simulink model "Target_Control_System"  (R2021b)
settings: Solver=FixedStepDiscrete  StartTime=0.0  StopTime=5  RelTol=1e-3
PreLoadFcn:
  | RTWConfigurationCB('preloadfcn', bdroot);
PostLoadFcn:
  | load('configuration/data_struct.mat');
  | load('configuration/fluxMaps_propMotor.mat');
  | load('configuration/parameterInit_PROP.mat');
  | load('configuration/parameterInit_PUMP.mat');
  | load('configuration/parameterInit_PITCH.mat');
  | load('configuration/parameterInit_TILT.mat');
  | %load('configuration/base_workspace_signal_definition.mat');
  | %load('resolvedatastores_to_baseworkspace_for_faster_simulation.mat');
model workspace (MAT data in the model file):
  SIMULATION_OPTIONS : Simulink.Parameter (value not decoded)
  TARGET_CODE_GEN : Simulink.Parameter (value not decoded)
  TCS_SAMPLE_FREQ_HZ : Simulink.Parameter (value not decoded)
symbols that are objects in the model workspace (value not decoded): TARGET_CODE_GEN, TCS_SAMPLE_FREQ_HZ
undefined symbols (not defined in the file): A_DQ_REF_LPF_INIT__PITCH, A_DQ_REF_LPF_INIT__PROP, A_DQ_REF_LPF_INIT__PUMP, A_DQ_REF_LPF_INIT__TILT, A_OBSERVER_CONFIDENCE_INIT__PITCH, A_OBSERVER_CONFIDENCE_INIT__PROP, A_OBSERVER_CONFIDENCE_INIT__PUMP, A_OBSERVER_CONFIDENCE_INIT__TILT, ACTUATOR_MAX_ANGLE_TRIP__PITCH, ACTUATOR_MIN_ANGLE_TRIP__PITCH, ACTUATOR_POS_SENSOR_INV_DIRECTION__PITCH, ACTUATOR_POS_SENSOR_INV_DIRECTION__TILT, ACTUATOR_POS_SENSOR_OFFSET__PITCH, ACTUATOR_POS_SENSOR_OFFSET__TILT, ADC_scaler1_baseaddr_TILT, ADC_SCALER_FLOAT_TO_FIXPOINT_EXPANSION, ANGLE_ELEC_FROM_SENSOR_OFFSET_INIT__PITCH, ANGLE_ELEC_FROM_SENSOR_OFFSET_INIT__PROP, ANGLE_ELEC_FROM_SENSOR_OFFSET_INIT__PUMP, ANGLE_ELEC_FROM_SENSOR_OFFSET_INIT__TILT, AUTO_CLEAR_FAULTS_ENABLED__PITCH, AUTO_CLEAR_FAULTS_ENABLED__PROP, AUTO_CLEAR_FAULTS_ENABLED__PUMP, AUTO_CLEAR_FAULTS_ENABLED__TILT, AUTO_CLEAR_FAULTS_WAIT_TICKS__PITCH, AUTO_CLEAR_FAULTS_WAIT_TICKS__PROP, AUTO_CLEAR_FAULTS_WAIT_TICKS__PUMP, AUTO_CLEAR_FAULTS_WAIT_TICKS__TILT, AUTO_I_ZERO_IDLE_TICKS__PITCH, AUTO_I_ZERO_IDLE_TICKS__PROP, AUTO_I_ZERO_IDLE_TICKS__PUMP, AUTO_I_ZERO_IDLE_TICKS__TILT, AUTO_I_ZERO_OFFSET_IDC_THRESHOLD__PITCH, AUTO_I_ZERO_OFFSET_IDC_THRESHOLD__PROP, AUTO_I_ZERO_OFFSET_IDC_THRESHOLD__PUMP, AUTO_I_ZERO_OFFSET_IDC_THRESHOLD__TILT, AUTO_I_ZERO_OFFSET_IPH_THRESHOLD__PITCH, AUTO_I_ZERO_OFFSET_IPH_THRESHOLD__PROP, AUTO_I_ZERO_OFFSET_IPH_THRESHOLD__PUMP, AUTO_I_ZERO_OFFSET_IPH_THRESHOLD__TILT, AUTO_SENSORLESS_SWITCHOVER_DISABLE_OMEGA, AUTO_SENSORLESS_SWITCHOVER_ENABLE_OMEGA, AUTO_SENSORLESS_SWITCHOVER_MIN_CONFIDENCE, AUXILIARY_PROTECTION_UNIT_BASEADDR__TILT, blanking_max_error_omega_INIT_PITCH, blanking_max_error_omega_INIT_TILT, blanking_max_error_position_INIT_PITCH, blanking_max_error_position_INIT_TILT, BRUTE_START_I_Q_REF_RAMP_SPEED__PITCH, BRUTE_START_I_Q_REF_RAMP_SPEED__PROP, BRUTE_START_I_Q_REF_RAMP_SPEED__PUMP, BRUTE_START_I_Q_REF_RAMP_SPEED__TILT, CONTROL_LOOP_DT_INIT__PITCH, CONTROL_LOOP_DT_INIT__PROP, CONTROL_LOOP_DT_INIT__PUMP, CONTROL_LOOP_DT_INIT__TILT, CORRECTION_FILTER_SCALE__PITCH, CORRECTION_FILTER_SCALE__PROP, CORRECTION_FILTER_SCALE__PUMP, CORRECTION_FILTER_SCALE__TILT ... (+458)
libraries: simulink x178, Reusables_Lib x24
(part 4 of 47)

== system Target_Control_System/Target_Control_System/InterruptFunction/pumpMotor_dataToIsr ==
  motorDataFromMainToIsr : TriggerPort  TriggerType=function-call  VariantControl=Variant
  Data Store Read : DataStoreRead  DataStoreName=oPump  DataStoreElements=oPump.oMot_.oOut_.fOneOverUdc_  IndexOptions=Index vector (dialog)  Indices=1  OutputSizes=1
  Data Store Read1 : DataStoreRead  DataStoreName=oPump  DataStoreElements=oPump.oMot_.oState_.oRampDataOmegaERef_.fRampOut_  IndexOptions=Index vector (dialog)  Indices=1  OutputSizes=1
  Data Store Read10 : DataStoreRead  DataStoreName=oPump  DataStoreElements=oPump.oMot_.oOut_.uiCurrentControllerActive_  IndexOptions=Index vector (dialog)  Indices=1  OutputSizes=1
  Data Store Read11 : DataStoreRead  DataStoreName=oPump  DataStoreElements=oPump.oMot_.oState_.oRampDataFluxFeedforwardGain_.fRampOut_  IndexOptions=Index vector (dialog)  Indices=1  OutputSizes=1
  Data Store Read12 : DataStoreRead  DataStoreName=oPump  DataStoreElements=oPump.oMot_.oState_.uiDriveState_  IndexOptions=Index vector (dialog)  Indices=1  OutputSizes=1
  Data Store Read13 : DataStoreRead  DataStoreName=oPump  DataStoreElements=oPump.oMot_.oOut_.uiPwmRequestFromMain_  IndexOptions=Index vector (dialog)  Indices=1  OutputSizes=1
  Data Store Read14 : DataStoreRead  DataStoreName=oPump  DataStoreElements=oPump.oMot_.oOut_.uiPwmDutyTicksFromMainA_  IndexOptions=Index vector (dialog)  Indices=1  OutputSizes=1
  Data Store Read15 : DataStoreRead  DataStoreName=oPump  DataStoreElements=oPump.oMot_.oOut_.uiPwmDutyTicksFromMainB_  IndexOptions=Index vector (dialog)  Indices=1  OutputSizes=1
  Data Store Read16 : DataStoreRead  DataStoreName=oPump  DataStoreElements=oPump.oMot_.oOut_.uiPwmDutyTicksFromMainC_  IndexOptions=Index vector (dialog)  Indices=1  OutputSizes=1
  Data Store Read17 : DataStoreRead  DataStoreName=oPump  DataStoreElements=oPump.oMot_.oState_.oPosSensor_.fAngleElecFromSensor_  IndexOptions=Index vector (dialog)  Indices=1  OutputSizes=1
  Data Store Read18 : DataStoreRead  DataStoreName=oPump  DataStoreElements=oPump.oMot_.oState_.oPosSensor_.fOmegaEFromSensor_  IndexOptions=Index vector (dialog)  Indices=1  OutputSizes=1
  Data Store Read2 : DataStoreRead  DataStoreName=oPump  DataStoreElements=oPump.oMot_.oState_.oRampDataFluxMasterAngleOffset_.fRampOut_  IndexOptions=Index vector (dialog)  Indices=1  OutputSizes=1
  Data Store Read3 : DataStoreRead  DataStoreName=oPump  DataStoreElements=oPump.oMot_.oState_.oRampDataIqRef_.fRampOut_  IndexOptions=Index vector (dialog)  Indices=1  OutputSizes=1
  Data Store Read4 : DataStoreRead  DataStoreName=oPump  DataStoreElements=oPump.oMot_.oState_.oRampDataIdRef_.fRampOut_  IndexOptions=Index vector (dialog)  Indices=1  OutputSizes=1
  Data Store Read5 : DataStoreRead  DataStoreName=oPump  DataStoreElements=oPump.oMot_.oParam_.fIdRefFractionOfIq_  IndexOptions=Index vector (dialog)  Indices=1  OutputSizes=1
  Data Store Read6 : DataStoreRead  DataStoreName=oPump  DataStoreElements=oPump.oMot_.oOut_.fUphFilterAmplitudeRatio_  IndexOptions=Index vector (dialog)  Indices=1  OutputSizes=1
  Data Store Read7 : DataStoreRead  DataStoreName=oPump  DataStoreElements=oPump.oMot_.oOut_.fUphFilterDelayAngleRad_  IndexOptions=Index vector (dialog)  Indices=1  OutputSizes=1
  Data Store Read8 : DataStoreRead  DataStoreName=oPump  DataStoreElements=oPump.oMot_.oState_.oRampDataFluxMstrAngFrcd2clsdSmoothn_.fRampOut_  IndexOptions=Index vector (dialog)  Indices=1  OutputSizes=1
  Data Store Read9 : DataStoreRead  DataStoreName=oPump  DataStoreElements=oPump.oMot_.oOut_.uiForcedAngle_  IndexOptions=Index vector (dialog)  Indices=1  OutputSizes=1
  Data Store Write1 : DataStoreWrite  DataStoreName=oPump  DataStoreElements=oPump.oIsr_.oIn_.fOneOverUdc_  IndexOptions=Index vector (dialog)  Indices=1  OutputSizes=1
  Data Store Write10 : DataStoreWrite  DataStoreName=oPump  DataStoreElements=oPump.oIsr_.oIn_.uiForcedAngle_  IndexOptions=Index vector (dialog)  Indices=1  OutputSizes=1
  Data Store Write11 : DataStoreWrite  DataStoreName=oPump  DataStoreElements=oPump.oIsr_.oIn_.uiCurrentControllerActive_  IndexOptions=Index vector (dialog)  Indices=1  OutputSizes=1
  Data Store Write12 : DataStoreWrite  DataStoreName=oPump  DataStoreElements=oPump.oIsr_.oIn_.fFluxFeedforwardGainRampOut_  IndexOptions=Index vector (dialog)  Indices=1  OutputSizes=1
  Data Store Write13 : DataStoreWrite  DataStoreName=oPump  DataStoreElements=oPump.oIsr_.oIn_.uiDriveState_  IndexOptions=Index vector (dialog)  Indices=1  OutputSizes=1
  Data Store Write14 : DataStoreWrite  DataStoreName=oPump  DataStoreElements=oPump.oIsr_.oIn_.uiPwmRequestFromMain_  IndexOptions=Index vector (dialog)  Indices=1  OutputSizes=1
  Data Store Write15 : DataStoreWrite  DataStoreName=oPump  DataStoreElements=oPump.oIsr_.oIn_.uiPwmDutyTicksFromMainA_  IndexOptions=Index vector (dialog)  Indices=1  OutputSizes=1
  Data Store Write16 : DataStoreWrite  DataStoreName=oPump  DataStoreElements=oPump.oIsr_.oIn_.uiPwmDutyTicksFromMainB_  IndexOptions=Index vector (dialog)  Indices=1  OutputSizes=1
  Data Store Write17 : DataStoreWrite  DataStoreName=oPump  DataStoreElements=oPump.oIsr_.oIn_.uiPwmDutyTicksFromMainC_  IndexOptions=Index vector (dialog)  Indices=1  OutputSizes=1
  Data Store Write18 : DataStoreWrite  DataStoreName=oPump  DataStoreElements=oPump.oIsr_.oIn_.fAngleElecFromPosSensor_  IndexOptions=Index vector (dialog)  Indices=1  OutputSizes=1
  Data Store Write19 : DataStoreWrite  DataStoreName=oPump  DataStoreElements=oPump.oIsr_.oIn_.fOmegaElecFromPosSensor_  IndexOptions=Index vector (dialog)  Indices=1  OutputSizes=1
  Data Store Write2 : DataStoreWrite  DataStoreName=oPump  DataStoreElements=oPump.oIsr_.oIn_.fOmegaERefRampOut_  IndexOptions=Index vector (dialog)  Indices=1  OutputSizes=1
  Data Store Write3 : DataStoreWrite  DataStoreName=oPump  DataStoreElements=oPump.oIsr_.oIn_.fFluxMasterAngleOffsetRampOut_  IndexOptions=Index vector (dialog)  Indices=1  OutputSizes=1
  Data Store Write4 : DataStoreWrite  DataStoreName=oPump  DataStoreElements=oPump.oIsr_.oIn_.fIqRefRampOut_  IndexOptions=Index vector (dialog)  Indices=1  OutputSizes=1
  Data Store Write5 : DataStoreWrite  DataStoreName=oPump  DataStoreElements=oPump.oIsr_.oIn_.fIdRefRampOut_  IndexOptions=Index vector (dialog)  Indices=1  OutputSizes=1
  Data Store Write6 : DataStoreWrite  DataStoreName=oPump  DataStoreElements=oPump.oIsr_.oIn_.fIdRefFractionOfIq_  IndexOptions=Index vector (dialog)  Indices=1  OutputSizes=1
  Data Store Write7 : DataStoreWrite  DataStoreName=oPump  DataStoreElements=oPump.oIsr_.oIn_.fUphFilterAmplitudeRatio_  IndexOptions=Index vector (dialog)  Indices=1  OutputSizes=1
  Data Store Write8 : DataStoreWrite  DataStoreName=oPump  DataStoreElements=oPump.oIsr_.oIn_.fUphFilterDelayAngleRad_  IndexOptions=Index vector (dialog)  Indices=1  OutputSizes=1
  Data Store Write9 : DataStoreWrite  DataStoreName=oPump  DataStoreElements=oPump.oIsr_.oIn_.fFluxMasterAngleForced2closedSmoothingRampOut_  IndexOptions=Index vector (dialog)  Indices=1  OutputSizes=1
  wires:
  Data Store Read2/1 -> Data Store Write3/1
  Data Store Read12/1 -> Data Store Write13/1
  Data Store Read13/1 -> Data Store Write14/1
  Data Store Read16/1 -> Data Store Write17/1
  Data Store Read5/1 -> Data Store Write6/1
  Data Store Read10/1 -> Data Store Write11/1
  Data Store Read/1 -> Data Store Write1/1
  Data Store Read14/1 -> Data Store Write15/1
  Data Store Read8/1 -> Data Store Write9/1
  Data Store Read9/1 -> Data Store Write10/1
  Data Store Read3/1 -> Data Store Write4/1
  Data Store Read7/1 -> Data Store Write8/1
  Data Store Read11/1 -> Data Store Write12/1
  Data Store Read15/1 -> Data Store Write16/1
  Data Store Read17/1 -> Data Store Write18/1
  Data Store Read1/1 -> Data Store Write2/1
  Data Store Read18/1 -> Data Store Write19/1
  Data Store Read4/1 -> Data Store Write5/1
  Data Store Read6/1 -> Data Store Write7/1

== system Target_Control_System/Target_Control_System/InterruptFunction/pumpMotor_dataToMain ==
  motorDataFromIsrToMain : TriggerPort  TriggerType=function-call  VariantControl=Variant
  Constant : Constant  OutDataTypeStr=uint32  SampleTime=-1
  Data Store Read : DataStoreRead  DataStoreName=oPump  DataStoreElements=oPump.oIsr_.oOut_.fPowerDc_  IndexOptions=Index vector (dialog)  Indices=1  OutputSizes=1
  Data Store Read1 : DataStoreRead  DataStoreName=oPump  DataStoreElements=oPump.oIsr_.oOut_.fTEstimate_  IndexOptions=Index vector (dialog)  Indices=1  OutputSizes=1
  Data Store Read10 : DataStoreRead  DataStoreName=oPump  DataStoreElements=oPump.oIsr_.oState_.fUdRef_  IndexOptions=Index vector (dialog)  Indices=1  OutputSizes=1
  Data Store Read11 : DataStoreRead  DataStoreName=oPump  DataStoreElements=oPump.oIsr_.oState_.fFluxMasterAngle_  IndexOptions=Index vector (dialog)  Indices=1  OutputSizes=1
  Data Store Read12 : DataStoreRead  DataStoreName=oPump  DataStoreElements=oPump.oIsr_.oState_.fSoftILimitActual_  IndexOptions=Index vector (dialog)  Indices=1  OutputSizes=1
  Data Store Read13 : DataStoreRead  DataStoreName=oPump  DataStoreElements=oPump.oIsr_.oState_.fFluxMainAngleRaw2_  IndexOptions=Index vector (dialog)  Indices=1  OutputSizes=1
  Data Store Read14 : DataStoreRead  DataStoreName=oPump  DataStoreElements=oPump.oIsr_.oState_.fRMeasured_  IndexOptions=Index vector (dialog)  Indices=1  OutputSizes=1
  Data Store Read15 : DataStoreRead  DataStoreName=oPump  DataStoreElements=oPump.oIsr_.oOut_.uiPwmSetByIsr_  IndexOptions=Index vector (dialog)  Indices=1  OutputSizes=1
  Data Store Read16 : DataStoreRead  DataStoreName=oPump  DataStoreElements=oPump.oIsr_.oIn_.oAdcData_.fIa_  IndexOptions=Index vector (dialog)  Indices=1  OutputSizes=1
  Data Store Read17 : DataStoreRead  DataStoreName=oPump  DataStoreElements=oPump.oIsr_.oIn_.oAdcData_.fIb_  IndexOptions=Index vector (dialog)  Indices=1  OutputSizes=1
  Data Store Read18 : DataStoreRead  DataStoreName=oPump  DataStoreElements=oPump.oIsr_.oIn_.oAdcData_.fIc_  IndexOptions=Index vector (dialog)  Indices=1  OutputSizes=1
  Data Store Read19 : DataStoreRead  DataStoreName=oPump  DataStoreElements=oPump.oIsr_.oIn_.oAdcData_.fIdc_  IndexOptions=Index vector (dialog)  Indices=1  OutputSizes=1
  Data Store Read2 : DataStoreRead  DataStoreName=oPump  DataStoreElements=oPump.oIsr_.oOut_.fIPhaseMagnitude_  IndexOptions=Index vector (dialog)  Indices=1  OutputSizes=1
  Data Store Read20 : DataStoreRead  DataStoreName=oPump  DataStoreElements=oPump.oIsr_.oOut_.fUdc_  IndexOptions=Index vector (dialog)  Indices=1  OutputSizes=1
  Data Store Read21 : DataStoreRead  DataStoreName=oPump  DataStoreElements=oPump.oIsr_.oIn_.oAdcData_.fMotorEncoderFloat_  IndexOptions=Index vector (dialog)  Indices=1  OutputSizes=1
  Data Store Read22 : DataStoreRead  DataStoreName=oPump  DataStoreElements=oPump.oIsr_.oIn_.oAdcData_.fOutputEncoderFloat_  IndexOptions=Index vector (dialog)  Indices=1  OutputSizes=1
  Data Store Read23 : DataStoreRead  DataStoreName=oPump  DataStoreElements=oPump.oIsr_.oIn_.oAdcData_.fMotorSensorSpeed_  IndexOptions=Index vector (dialog)  Indices=1  OutputSizes=1
  Data Store Read3 : DataStoreRead  DataStoreName=oPump  DataStoreElements=oPump.oIsr_.oState_.fFluxMainMagnitudeLpf_  IndexOptions=Index vector (dialog)  Indices=1  OutputSizes=1
  Data Store Read4 : DataStoreRead  DataStoreName=oPump  DataStoreElements=oPump.oIsr_.oState_.fOmegaEObserverLpf2_  IndexOptions=Index vector (dialog)  Indices=1  OutputSizes=1
  Data Store Read5 : DataStoreRead  DataStoreName=oPump  DataStoreElements=oPump.oIsr_.oState_.fOmegaEObserverRaw2_  IndexOptions=Index vector (dialog)  Indices=1  OutputSizes=1
  Data Store Read6 : DataStoreRead  DataStoreName=oPump  DataStoreElements=oPump.oIsr_.oState_.fId_  IndexOptions=Index vector (dialog)  Indices=1  OutputSizes=1
  Data Store Read7 : DataStoreRead  DataStoreName=oPump  DataStoreElements=oPump.oIsr_.oState_.fIq_  IndexOptions=Index vector (dialog)  Indices=1  OutputSizes=1
  Data Store Read8 : DataStoreRead  DataStoreName=oPump  DataStoreElements=oPump.oIsr_.oState_.fIdRefTotal_  IndexOptions=Index vector (dialog)  Indices=1  OutputSizes=1
  Data Store Read9 : DataStoreRead  DataStoreName=oPump  DataStoreElements=oPump.oIsr_.oState_.fUqRef_  IndexOptions=Index vector (dialog)  Indices=1  OutputSizes=1
  Data Store Write1 : DataStoreWrite  DataStoreName=oPump  DataStoreElements=oPump.oMot_.oIn_.fPowerDc_  IndexOptions=Index vector (dialog)  Indices=1  OutputSizes=1
  Data Store Write10 : DataStoreWrite  DataStoreName=oPump  DataStoreElements=oPump.oMot_.oIn_.fUqRef_  IndexOptions=Index vector (dialog)  Indices=1  OutputSizes=1
  Data Store Write11 : DataStoreWrite  DataStoreName=oPump  DataStoreElements=oPump.oMot_.oIn_.fUdRef_  IndexOptions=Index vector (dialog)  Indices=1  OutputSizes=1
  Data Store Write12 : DataStoreWrite  DataStoreName=oPump  DataStoreElements=oPump.oMot_.oIn_.fFluxMasterAngle_  IndexOptions=Index vector (dialog)  Indices=1  OutputSizes=1
  Data Store Write13 : DataStoreWrite  DataStoreName=oPump  DataStoreElements=oPump.oMot_.oIn_.fSoftILimitActual_  IndexOptions=Index vector (dialog)  Indices=1  OutputSizes=1
  Data Store Write14 : DataStoreWrite  DataStoreName=oPump  DataStoreElements=oPump.oMot_.oIn_.fFluxMainAngleRaw2_  IndexOptions=Index vector (dialog)  Indices=1  OutputSizes=1
  Data Store Write15 : DataStoreWrite  DataStoreName=oPump  DataStoreElements=oPump.oMot_.oIn_.fRMeasured_  IndexOptions=Index vector (dialog)  Indices=1  OutputSizes=1
  Data Store Write16 : DataStoreWrite  DataStoreName=oPump  DataStoreElements=oPump.oMot_.oIn_.uiPwmSetByIsr_  IndexOptions=Index vector (dialog)  Indices=1  OutputSizes=1
  Data Store Write17 : DataStoreWrite  DataStoreName=oPump  DataStoreElements=oPump.oMot_.oIn_.oAdcData_.fIa_  IndexOptions=Index vector (dialog)  Indices=1  OutputSizes=1
  Data Store Write18 : DataStoreWrite  DataStoreName=oPump  DataStoreElements=oPump.oMot_.oIn_.oAdcData_.fIb_  IndexOptions=Index vector (dialog)  Indices=1  OutputSizes=1
  Data Store Write19 : DataStoreWrite  DataStoreName=oPump  DataStoreElements=oPump.oMot_.oIn_.oAdcData_.fIc_  IndexOptions=Index vector (dialog)  Indices=1  OutputSizes=1
  Data Store Write2 : DataStoreWrite  DataStoreName=oPump  DataStoreElements=oPump.oMot_.oIn_.fTEstimate_  IndexOptions=Index vector (dialog)  Indices=1  OutputSizes=1
  Data Store Write20 : DataStoreWrite  DataStoreName=oPump  DataStoreElements=oPump.oMot_.oIn_.oAdcData_.fIdc_  IndexOptions=Index vector (dialog)  Indices=1  OutputSizes=1
  Data Store Write21 : DataStoreWrite  DataStoreName=oPump  DataStoreElements=oPump.oMot_.oIn_.oAdcData_.fUdc_  IndexOptions=Index vector (dialog)  Indices=1  OutputSizes=1
  Data Store Write22 : DataStoreWrite  DataStoreName=oPump  DataStoreElements=oPump.oMot_.oIn_.oAdcData_.fMotorEncoderFloat_  IndexOptions=Index vector (dialog)  Indices=1  OutputSizes=1
  Data Store Write23 : DataStoreWrite  DataStoreName=oPump  DataStoreElements=oPump.oMot_.oIn_.oAdcData_.fOutputEncoderFloat_  IndexOptions=Index vector (dialog)  Indices=1  OutputSizes=1
  Data Store Write24 : DataStoreWrite  DataStoreName=oPump  DataStoreElements=oPump.oMot_.oIn_.oAdcData_.fMotorSensorSpeed_  IndexOptions=Index vector (dialog)  Indices=1  OutputSizes=1
  Data Store Write25 : DataStoreWrite  DataStoreName=oPump  DataStoreElements=oPump.oMot_.oIn_.uiDataFromIsrToMainUpdated_  IndexOptions=Index vector (dialog)  Indices=1  OutputSizes=1
  Data Store Write3 : DataStoreWrite  DataStoreName=oPump  DataStoreElements=oPump.oMot_.oIn_.fIPhaseMagnitude_  IndexOptions=Index vector (dialog)  Indices=1  OutputSizes=1
  Data Store Write4 : DataStoreWrite  DataStoreName=oPump  DataStoreElements=oPump.oMot_.oIn_.fFluxMainMagnitudeLpf_  IndexOptions=Index vector (dialog)  Indices=1  OutputSizes=1
  Data Store Write5 : DataStoreWrite  DataStoreName=oPump  DataStoreElements=oPump.oMot_.oIn_.fOmegaEObserverLpf2_  IndexOptions=Index vector (dialog)  Indices=1  OutputSizes=1
  Data Store Write6 : DataStoreWrite  DataStoreName=oPump  DataStoreElements=oPump.oMot_.oIn_.fOmegaEObserverRaw2_  IndexOptions=Index vector (dialog)  Indices=1  OutputSizes=1
  Data Store Write7 : DataStoreWrite  DataStoreName=oPump  DataStoreElements=oPump.oMot_.oIn_.fId_  IndexOptions=Index vector (dialog)  Indices=1  OutputSizes=1
  Data Store Write8 : DataStoreWrite  DataStoreName=oPump  DataStoreElements=oPump.oMot_.oIn_.fIq_  IndexOptions=Index vector (dialog)  Indices=1  OutputSizes=1
  Data Store Write9 : DataStoreWrite  DataStoreName=oPump  DataStoreElements=oPump.oMot_.oIn_.fIdRefTotal_  IndexOptions=Index vector (dialog)  Indices=1  OutputSizes=1
  wires:
  Data Store Read21/1 -> Data Store Write22/1
  Data Store Read19/1 -> Data Store Write20/1
  Data Store Read3/1 -> Data Store Write4/1
  Data Store Read20/1 -> Data Store Write21/1
  Data Store Read23/1 -> Data Store Write24/1
  Constant/1 -> Data Store Write25/1
  Data Store Read9/1 -> Data Store Write10/1
  Data Store Read22/1 -> Data Store Write23/1
  Data Store Read14/1 -> Data Store Write15/1
  Data Store Read7/1 -> Data Store Write8/1
  Data Store Read/1 -> Data Store Write1/1
  Data Store Read16/1 -> Data Store Write17/1
  Data Store Read10/1 -> Data Store Write11/1
  Data Store Read4/1 -> Data Store Write5/1
  Data Store Read12/1 -> Data Store Write13/1
  Data Store Read5/1 -> Data Store Write6/1
  Data Store Read8/1 -> Data Store Write9/1
  Data Store Read17/1 -> Data Store Write18/1
  Data Store Read2/1 -> Data Store Write3/1
  Data Store Read6/1 -> Data Store Write7/1
  Data Store Read13/1 -> Data Store Write14/1
  Data Store Read11/1 -> Data Store Write12/1
  Data Store Read1/1 -> Data Store Write2/1
  Data Store Read15/1 -> Data Store Write16/1
  Data Store Read18/1 -> Data Store Write19/1

== system Target_Control_System/Target_Control_System/InterruptFunction/pumpMotor_isrSchedule ==
  FunctionCallSchedulePump : TriggerPort  TriggerType=function-call  VariantControl=Variant
  Constant : Constant  OutDataTypeStr=uint32  SampleTime=-1
  Constant1 : Constant  Value=3  OutDataTypeStr=uint32  SampleTime=-1
  Data Store Read : DataStoreRead  DataStoreName=mdl_suiIsrSmallInvCounter_  IndexOptions=Index vector (dialog)  Indices=1  OutputSizes=1
  Equal : RelationalOperator  Operator===  OutDataTypeStr=boolean  RndMeth=Simplest
  Equal1 : RelationalOperator  Operator===  OutDataTypeStr=boolean  RndMeth=Simplest
  OR : Logic  Operator=OR  AllPortsSameDT=off  OutDataTypeStr=boolean
  Triggered Subsystem : Subsystem  TreatAsAtomicUnit=on
  Output : Outport
  wires:
  Constant1/1 -> Equal1/2
  Equal1/1 -> OR/2
  Constant/1 -> Equal/1
  Data Store Read/1 -> Equal1/1, Equal/2
  Equal/1 -> OR/1
  Triggered Subsystem/1(Output) -> Output/1
  OR/1 -> Triggered Subsystem/Trigger

== system Target_Control_System/Target_Control_System/InterruptFunction/pumpMotor_isrTask ==
  motorIntTaskStep : TriggerPort  TriggerType=function-call  VariantControl=Variant  PortDimensions=1
  Function-Call Generator : simulink/Ports & Subsystems/Function-Call Generator  sample_time=-1  numberOfIterations=1  DisallowWideOutput=off
  Function-Call Split{1..8} (8 alike) : FunctionCallSplit  NumOutputPorts=2
  abcToAlphaBeta : Subsystem  TreatAsAtomicUnit=on
  currentController : Subsystem  TreatAsAtomicUnit=on
  dqTransform : Subsystem  TreatAsAtomicUnit=on
  fluxAngleCalculations : Subsystem  TreatAsAtomicUnit=on
  fluxObserver : Subsystem  TreatAsAtomicUnit=on
  isrStateMachine : Subsystem  TreatAsAtomicUnit=on
  pwmGeneration : Subsystem  TreatAsAtomicUnit=on
  resetFlags : Subsystem  TreatAsAtomicUnit=on
  softCurrentLimiting : Subsystem  TreatAsAtomicUnit=on
  wires:
  Function-Call Split8/2 -> isrStateMachine/Trigger
  Function-Call Split8/1 -> pwmGeneration/Trigger
  Function-Call Split7/2 -> Function-Call Split8/1
  Function-Call Split7/1 -> currentController/Trigger
  Function-Call Split1/2 -> Function-Call Split7/1
  Function-Call Split1/1 -> dqTransform/Trigger
  Function-Call Split6/2 -> Function-Call Split1/1
  Function-Call Split6/1 -> fluxAngleCalculations/Trigger
  Function-Call Split5/2 -> Function-Call Split6/1
  Function-Call Split5/1 -> fluxObserver/Trigger
  Function-Call Split4/2 -> Function-Call Split5/1
  Function-Call Split4/1 -> abcToAlphaBeta/Trigger
  Function-Call Split3/2 -> Function-Call Split4/1
  Function-Call Split3/1 -> softCurrentLimiting/Trigger
  Function-Call Split2/2 -> Function-Call Split3/1
  Function-Call Split2/1 -> resetFlags/Trigger
  Function-Call Generator/1 -> Function-Call Split2/1

== system Target_Control_System/Target_Control_System/InterruptFunction/pumpMotor_setPwm ==
  setPwmDuty : TriggerPort  TriggerType=function-call  VariantControl=Variant
  Data Store Read1 : DataStoreRead  DataStoreName=oPump  DataStoreElements=oPump.oIsr_.oState_.iPwmUpdated_  IndexOptions=Index vector (dialog)  Indices=1  OutputSizes=1
  ModelSourceFPGAPump : Subsystem  Variant=on
  NOT : Logic  Operator=NOT  AllPortsSameDT=off  OutDataTypeStr=boolean
  Subsystem : Subsystem
  wires:
  NOT/1 -> Subsystem/Enable
  Data Store Read1/1 -> NOT/1

== system Target_Control_System/Target_Control_System/InterruptFunction/tiltMotor_dataToIsr ==
  motorDataFromMainToIsr : TriggerPort  TriggerType=function-call  VariantControl=Variant
  Data Store Read : DataStoreRead  DataStoreName=oTilt  DataStoreElements=oTilt.oMot_.oOut_.fOneOverUdc_  IndexOptions=Index vector (dialog)  Indices=1  OutputSizes=1
  Data Store Read1 : DataStoreRead  DataStoreName=oTilt  DataStoreElements=oTilt.oMot_.oState_.oRampDataOmegaERef_.fRampOut_  IndexOptions=Index vector (dialog)  Indices=1  OutputSizes=1
  Data Store Read10 : DataStoreRead  DataStoreName=oTilt  DataStoreElements=oTilt.oMot_.oOut_.uiCurrentControllerActive_  IndexOptions=Index vector (dialog)  Indices=1  OutputSizes=1
  Data Store Read11 : DataStoreRead  DataStoreName=oTilt  DataStoreElements=oTilt.oMot_.oState_.oRampDataFluxFeedforwardGain_.fRampOut_  IndexOptions=Index vector (dialog)  Indices=1  OutputSizes=1
  Data Store Read12 : DataStoreRead  DataStoreName=oTilt  DataStoreElements=oTilt.oMot_.oState_.uiDriveState_  IndexOptions=Index vector (dialog)  Indices=1  OutputSizes=1
  Data Store Read13 : DataStoreRead  DataStoreName=oTilt  DataStoreElements=oTilt.oMot_.oOut_.uiPwmRequestFromMain_  IndexOptions=Index vector (dialog)  Indices=1  OutputSizes=1
  Data Store Read14 : DataStoreRead  DataStoreName=oTilt  DataStoreElements=oTilt.oMot_.oOut_.uiPwmDutyTicksFromMainA_  IndexOptions=Index vector (dialog)  Indices=1  OutputSizes=1
  Data Store Read15 : DataStoreRead  DataStoreName=oTilt  DataStoreElements=oTilt.oMot_.oOut_.uiPwmDutyTicksFromMainB_  IndexOptions=Index vector (dialog)  Indices=1  OutputSizes=1
  Data Store Read16 : DataStoreRead  DataStoreName=oTilt  DataStoreElements=oTilt.oMot_.oOut_.uiPwmDutyTicksFromMainC_  IndexOptions=Index vector (dialog)  Indices=1  OutputSizes=1
  Data Store Read17 : DataStoreRead  DataStoreName=oTilt  DataStoreElements=oTilt.oMot_.oState_.oPosSensor_.fAngleElecFromSensor_  IndexOptions=Index vector (dialog)  Indices=1  OutputSizes=1
  Data Store Read18 : DataStoreRead  DataStoreName=oTilt  DataStoreElements=oTilt.oMot_.oState_.oPosSensor_.fOmegaEFromSensor_  IndexOptions=Index vector (dialog)  Indices=1  OutputSizes=1
  Data Store Read2 : DataStoreRead  DataStoreName=oTilt  DataStoreElements=oTilt.oMot_.oState_.oRampDataFluxMasterAngleOffset_.fRampOut_  IndexOptions=Index vector (dialog)  Indices=1  OutputSizes=1
  Data Store Read3 : DataStoreRead  DataStoreName=oTilt  DataStoreElements=oTilt.oMot_.oState_.oRampDataIqRef_.fRampOut_  IndexOptions=Index vector (dialog)  Indices=1  OutputSizes=1
  Data Store Read4 : DataStoreRead  DataStoreName=oTilt  DataStoreElements=oTilt.oMot_.oState_.oRampDataIdRef_.fRampOut_  IndexOptions=Index vector (dialog)  Indices=1  OutputSizes=1
  Data Store Read5 : DataStoreRead  DataStoreName=oTilt  DataStoreElements=oTilt.oMot_.oParam_.fIdRefFractionOfIq_  IndexOptions=Index vector (dialog)  Indices=1  OutputSizes=1
  Data Store Read6 : DataStoreRead  DataStoreName=oTilt  DataStoreElements=oTilt.oMot_.oOut_.fUphFilterAmplitudeRatio_  IndexOptions=Index vector (dialog)  Indices=1  OutputSizes=1
  Data Store Read7 : DataStoreRead  DataStoreName=oTilt  DataStoreElements=oTilt.oMot_.oOut_.fUphFilterDelayAngleRad_  IndexOptions=Index vector (dialog)  Indices=1  OutputSizes=1
  Data Store Read8 : DataStoreRead  DataStoreName=oTilt  DataStoreElements=oTilt.oMot_.oState_.oRampDataFluxMstrAngFrcd2clsdSmoothn_.fRampOut_  IndexOptions=Index vector (dialog)  Indices=1  OutputSizes=1
  Data Store Read9 : DataStoreRead  DataStoreName=oTilt  DataStoreElements=oTilt.oMot_.oOut_.uiForcedAngle_  IndexOptions=Index vector (dialog)  Indices=1  OutputSizes=1
  Data Store Write1 : DataStoreWrite  DataStoreName=oTilt  DataStoreElements=oTilt.oIsr_.oIn_.fOneOverUdc_  IndexOptions=Index vector (dialog)  Indices=1  OutputSizes=1
  Data Store Write10 : DataStoreWrite  DataStoreName=oTilt  DataStoreElements=oTilt.oIsr_.oIn_.uiForcedAngle_  IndexOptions=Index vector (dialog)  Indices=1  OutputSizes=1
  Data Store Write11 : DataStoreWrite  DataStoreName=oTilt  DataStoreElements=oTilt.oIsr_.oIn_.uiCurrentControllerActive_  IndexOptions=Index vector (dialog)  Indices=1  OutputSizes=1
  Data Store Write12 : DataStoreWrite  DataStoreName=oTilt  DataStoreElements=oTilt.oIsr_.oIn_.fFluxFeedforwardGainRampOut_  IndexOptions=Index vector (dialog)  Indices=1  OutputSizes=1
  Data Store Write13 : DataStoreWrite  DataStoreName=oTilt  DataStoreElements=oTilt.oIsr_.oIn_.uiDriveState_  IndexOptions=Index vector (dialog)  Indices=1  OutputSizes=1
  Data Store Write14 : DataStoreWrite  DataStoreName=oTilt  DataStoreElements=oTilt.oIsr_.oIn_.uiPwmRequestFromMain_  IndexOptions=Index vector (dialog)  Indices=1  OutputSizes=1
  Data Store Write15 : DataStoreWrite  DataStoreName=oTilt  DataStoreElements=oTilt.oIsr_.oIn_.uiPwmDutyTicksFromMainA_  IndexOptions=Index vector (dialog)  Indices=1  OutputSizes=1
  Data Store Write16 : DataStoreWrite  DataStoreName=oTilt  DataStoreElements=oTilt.oIsr_.oIn_.uiPwmDutyTicksFromMainB_  IndexOptions=Index vector (dialog)  Indices=1  OutputSizes=1
  Data Store Write17 : DataStoreWrite  DataStoreName=oTilt  DataStoreElements=oTilt.oIsr_.oIn_.uiPwmDutyTicksFromMainC_  IndexOptions=Index vector (dialog)  Indices=1  OutputSizes=1
  Data Store Write18 : DataStoreWrite  DataStoreName=oTilt  DataStoreElements=oTilt.oIsr_.oIn_.fAngleElecFromPosSensor_  IndexOptions=Index vector (dialog)  Indices=1  OutputSizes=1
  Data Store Write19 : DataStoreWrite  DataStoreName=oTilt  DataStoreElements=oTilt.oIsr_.oIn_.fOmegaElecFromPosSensor_  IndexOptions=Index vector (dialog)  Indices=1  OutputSizes=1
  Data Store Write2 : DataStoreWrite  DataStoreName=oTilt  DataStoreElements=oTilt.oIsr_.oIn_.fOmegaERefRampOut_  IndexOptions=Index vector (dialog)  Indices=1  OutputSizes=1
  Data Store Write3 : DataStoreWrite  DataStoreName=oTilt  DataStoreElements=oTilt.oIsr_.oIn_.fFluxMasterAngleOffsetRampOut_  IndexOptions=Index vector (dialog)  Indices=1  OutputSizes=1
  Data Store Write4 : DataStoreWrite  DataStoreName=oTilt  DataStoreElements=oTilt.oIsr_.oIn_.fIqRefRampOut_  IndexOptions=Index vector (dialog)  Indices=1  OutputSizes=1
  Data Store Write5 : DataStoreWrite  DataStoreName=oTilt  DataStoreElements=oTilt.oIsr_.oIn_.fIdRefRampOut_  IndexOptions=Index vector (dialog)  Indices=1  OutputSizes=1
  Data Store Write6 : DataStoreWrite  DataStoreName=oTilt  DataStoreElements=oTilt.oIsr_.oIn_.fIdRefFractionOfIq_  IndexOptions=Index vector (dialog)  Indices=1  OutputSizes=1
  Data Store Write7 : DataStoreWrite  DataStoreName=oTilt  DataStoreElements=oTilt.oIsr_.oIn_.fUphFilterAmplitudeRatio_  IndexOptions=Index vector (dialog)  Indices=1  OutputSizes=1
  Data Store Write8 : DataStoreWrite  DataStoreName=oTilt  DataStoreElements=oTilt.oIsr_.oIn_.fUphFilterDelayAngleRad_  IndexOptions=Index vector (dialog)  Indices=1  OutputSizes=1
  Data Store Write9 : DataStoreWrite  DataStoreName=oTilt  DataStoreElements=oTilt.oIsr_.oIn_.fFluxMasterAngleForced2closedSmoothingRampOut_  IndexOptions=Index vector (dialog)  Indices=1  OutputSizes=1
  wires:
  Data Store Read7/1 -> Data Store Write8/1
  Data Store Read17/1 -> Data Store Write18/1
  Data Store Read12/1 -> Data Store Write13/1
  Data Store Read15/1 -> Data Store Write16/1
  Data Store Read2/1 -> Data Store Write3/1
  Data Store Read8/1 -> Data Store Write9/1
  Data Store Read/1 -> Data Store Write1/1
  Data Store Read4/1 -> Data Store Write5/1
  Data Store Read3/1 -> Data Store Write4/1
  Data Store Read6/1 -> Data Store Write7/1
  Data Store Read14/1 -> Data Store Write15/1
  Data Store Read5/1 -> Data Store Write6/1
  Data Store Read18/1 -> Data Store Write19/1
  Data Store Read13/1 -> Data Store Write14/1
  Data Store Read16/1 -> Data Store Write17/1
  Data Store Read1/1 -> Data Store Write2/1
  Data Store Read9/1 -> Data Store Write10/1
  Data Store Read10/1 -> Data Store Write11/1
  Data Store Read11/1 -> Data Store Write12/1

== system Target_Control_System/Target_Control_System/InterruptFunction/tiltMotor_dataToMain ==
  motorDataFromIsrToMain : TriggerPort  TriggerType=function-call  VariantControl=Variant
  Constant : Constant  OutDataTypeStr=uint32  SampleTime=-1
  Data Store Read : DataStoreRead  DataStoreName=oTilt  DataStoreElements=oTilt.oIsr_.oOut_.fPowerDc_  IndexOptions=Index vector (dialog)  Indices=1  OutputSizes=1
  Data Store Read1 : DataStoreRead  DataStoreName=oTilt  DataStoreElements=oTilt.oIsr_.oOut_.fTEstimate_  IndexOptions=Index vector (dialog)  Indices=1  OutputSizes=1
  Data Store Read10 : DataStoreRead  DataStoreName=oTilt  DataStoreElements=oTilt.oIsr_.oState_.fUdRef_  IndexOptions=Index vector (dialog)  Indices=1  OutputSizes=1
  Data Store Read11 : DataStoreRead  DataStoreName=oTilt  DataStoreElements=oTilt.oIsr_.oState_.fFluxMasterAngle_  IndexOptions=Index vector (dialog)  Indices=1  OutputSizes=1
  Data Store Read12 : DataStoreRead  DataStoreName=oTilt  DataStoreElements=oTilt.oIsr_.oState_.fSoftILimitActual_  IndexOptions=Index vector (dialog)  Indices=1  OutputSizes=1
  Data Store Read13 : DataStoreRead  DataStoreName=oTilt  DataStoreElements=oTilt.oIsr_.oState_.fFluxMainAngleRaw2_  IndexOptions=Index vector (dialog)  Indices=1  OutputSizes=1
  Data Store Read14 : DataStoreRead  DataStoreName=oTilt  DataStoreElements=oTilt.oIsr_.oState_.fRMeasured_  IndexOptions=Index vector (dialog)  Indices=1  OutputSizes=1
  Data Store Read15 : DataStoreRead  DataStoreName=oTilt  DataStoreElements=oTilt.oIsr_.oOut_.uiPwmSetByIsr_  IndexOptions=Index vector (dialog)  Indices=1  OutputSizes=1
  Data Store Read16 : DataStoreRead  DataStoreName=oTilt  DataStoreElements=oTilt.oIsr_.oIn_.oAdcData_.fIa_  IndexOptions=Index vector (dialog)  Indices=1  OutputSizes=1
  Data Store Read17 : DataStoreRead  DataStoreName=oTilt  DataStoreElements=oTilt.oIsr_.oIn_.oAdcData_.fIb_  IndexOptions=Index vector (dialog)  Indices=1  OutputSizes=1
  Data Store Read18 : DataStoreRead  DataStoreName=oTilt  DataStoreElements=oTilt.oIsr_.oIn_.oAdcData_.fIc_  IndexOptions=Index vector (dialog)  Indices=1  OutputSizes=1
  Data Store Read19 : DataStoreRead  DataStoreName=oTilt  DataStoreElements=oTilt.oIsr_.oIn_.oAdcData_.fIdc_  IndexOptions=Index vector (dialog)  Indices=1  OutputSizes=1
  Data Store Read2 : DataStoreRead  DataStoreName=oTilt  DataStoreElements=oTilt.oIsr_.oOut_.fIPhaseMagnitude_  IndexOptions=Index vector (dialog)  Indices=1  OutputSizes=1
  Data Store Read20 : DataStoreRead  DataStoreName=oTilt  DataStoreElements=oTilt.oIsr_.oIn_.oAdcData_.fUdc_  IndexOptions=Index vector (dialog)  Indices=1  OutputSizes=1
  Data Store Read21 : DataStoreRead  DataStoreName=oTilt  DataStoreElements=oTilt.oIsr_.oIn_.oAdcData_.fMotorEncoderFloat_  IndexOptions=Index vector (dialog)  Indices=1  OutputSizes=1
  Data Store Read22 : DataStoreRead  DataStoreName=oTilt  DataStoreElements=oTilt.oIsr_.oIn_.oAdcData_.fOutputEncoderFloat_  IndexOptions=Index vector (dialog)  Indices=1  OutputSizes=1
  Data Store Read23 : DataStoreRead  DataStoreName=oTilt  DataStoreElements=oTilt.oIsr_.oIn_.oAdcData_.fMotorSensorSpeed_  IndexOptions=Index vector (dialog)  Indices=1  OutputSizes=1
  Data Store Read3 : DataStoreRead  DataStoreName=oTilt  DataStoreElements=oTilt.oIsr_.oState_.fFluxMainMagnitudeLpf_  IndexOptions=Index vector (dialog)  Indices=1  OutputSizes=1
  Data Store Read4 : DataStoreRead  DataStoreName=oTilt  DataStoreElements=oTilt.oIsr_.oState_.fOmegaEObserverLpf2_  IndexOptions=Index vector (dialog)  Indices=1  OutputSizes=1
  Data Store Read5 : DataStoreRead  DataStoreName=oTilt  DataStoreElements=oTilt.oIsr_.oState_.fOmegaEObserverRaw2_  IndexOptions=Index vector (dialog)  Indices=1  OutputSizes=1
  Data Store Read6 : DataStoreRead  DataStoreName=oTilt  DataStoreElements=oTilt.oIsr_.oState_.fId_  IndexOptions=Index vector (dialog)  Indices=1  OutputSizes=1
  Data Store Read7 : DataStoreRead  DataStoreName=oTilt  DataStoreElements=oTilt.oIsr_.oState_.fIq_  IndexOptions=Index vector (dialog)  Indices=1  OutputSizes=1
  Data Store Read8 : DataStoreRead  DataStoreName=oTilt  DataStoreElements=oTilt.oIsr_.oState_.fIdRefTotal_  IndexOptions=Index vector (dialog)  Indices=1  OutputSizes=1
  Data Store Read9 : DataStoreRead  DataStoreName=oTilt  DataStoreElements=oTilt.oIsr_.oState_.fUqRef_  IndexOptions=Index vector (dialog)  Indices=1  OutputSizes=1
  Data Store Write : DataStoreWrite  DataStoreName=oTilt  DataStoreElements=oTilt.oMot_.oIn_.uiDataFromIsrToMainUpdated_  IndexOptions=Index vector (dialog)  Indices=1  OutputSizes=1
  Data Store Write1 : DataStoreWrite  DataStoreName=oTilt  DataStoreElements=oTilt.oMot_.oIn_.fPowerDc_  IndexOptions=Index vector (dialog)  Indices=1  OutputSizes=1
  Data Store Write10 : DataStoreWrite  DataStoreName=oTilt  DataStoreElements=oTilt.oMot_.oIn_.fUqRef_  IndexOptions=Index vector (dialog)  Indices=1  OutputSizes=1
  Data Store Write11 : DataStoreWrite  DataStoreName=oTilt  DataStoreElements=oTilt.oMot_.oIn_.fUdRef_  IndexOptions=Index vector (dialog)  Indices=1  OutputSizes=1
  Data Store Write12 : DataStoreWrite  DataStoreName=oTilt  DataStoreElements=oTilt.oMot_.oIn_.fFluxMasterAngle_  IndexOptions=Index vector (dialog)  Indices=1  OutputSizes=1
  Data Store Write13 : DataStoreWrite  DataStoreName=oTilt  DataStoreElements=oTilt.oMot_.oIn_.fSoftILimitActual_  IndexOptions=Index vector (dialog)  Indices=1  OutputSizes=1
  Data Store Write14 : DataStoreWrite  DataStoreName=oTilt  DataStoreElements=oTilt.oMot_.oIn_.fFluxMainAngleRaw2_  IndexOptions=Index vector (dialog)  Indices=1  OutputSizes=1
  Data Store Write15 : DataStoreWrite  DataStoreName=oTilt  DataStoreElements=oTilt.oMot_.oIn_.fRMeasured_  IndexOptions=Index vector (dialog)  Indices=1  OutputSizes=1
  Data Store Write16 : DataStoreWrite  DataStoreName=oTilt  DataStoreElements=oTilt.oMot_.oIn_.uiPwmSetByIsr_  IndexOptions=Index vector (dialog)  Indices=1  OutputSizes=1
  Data Store Write17 : DataStoreWrite  DataStoreName=oTilt  DataStoreElements=oTilt.oMot_.oIn_.oAdcData_.fIa_  IndexOptions=Index vector (dialog)  Indices=1  OutputSizes=1
  Data Store Write18 : DataStoreWrite  DataStoreName=oTilt  DataStoreElements=oTilt.oMot_.oIn_.oAdcData_.fIb_  IndexOptions=Index vector (dialog)  Indices=1  OutputSizes=1
  Data Store Write19 : DataStoreWrite  DataStoreName=oTilt  DataStoreElements=oTilt.oMot_.oIn_.oAdcData_.fIc_  IndexOptions=Index vector (dialog)  Indices=1  OutputSizes=1
  Data Store Write2 : DataStoreWrite  DataStoreName=oTilt  DataStoreElements=oTilt.oMot_.oIn_.fTEstimate_  IndexOptions=Index vector (dialog)  Indices=1  OutputSizes=1
  Data Store Write20 : DataStoreWrite  DataStoreName=oTilt  DataStoreElements=oTilt.oMot_.oIn_.oAdcData_.fIdc_  IndexOptions=Index vector (dialog)  Indices=1  OutputSizes=1
  Data Store Write21 : DataStoreWrite  DataStoreName=oTilt  DataStoreElements=oTilt.oMot_.oIn_.oAdcData_.fUdc_  IndexOptions=Index vector (dialog)  Indices=1  OutputSizes=1
  Data Store Write22 : DataStoreWrite  DataStoreName=oTilt  DataStoreElements=oTilt.oMot_.oIn_.oAdcData_.fMotorEncoderFloat_  IndexOptions=Index vector (dialog)  Indices=1  OutputSizes=1
  Data Store Write23 : DataStoreWrite  DataStoreName=oTilt  DataStoreElements=oTilt.oMot_.oIn_.oAdcData_.fOutputEncoderFloat_  IndexOptions=Index vector (dialog)  Indices=1  OutputSizes=1
  Data Store Write24 : DataStoreWrite  DataStoreName=oTilt  DataStoreElements=oTilt.oMot_.oIn_.oAdcData_.fMotorSensorSpeed_  IndexOptions=Index vector (dialog)  Indices=1  OutputSizes=1
  Data Store Write3 : DataStoreWrite  DataStoreName=oTilt  DataStoreElements=oTilt.oMot_.oIn_.fIPhaseMagnitude_  IndexOptions=Index vector (dialog)  Indices=1  OutputSizes=1
  Data Store Write4 : DataStoreWrite  DataStoreName=oTilt  DataStoreElements=oTilt.oMot_.oIn_.fFluxMainMagnitudeLpf_  IndexOptions=Index vector (dialog)  Indices=1  OutputSizes=1
  Data Store Write5 : DataStoreWrite  DataStoreName=oTilt  DataStoreElements=oTilt.oMot_.oIn_.fOmegaEObserverLpf2_  IndexOptions=Index vector (dialog)  Indices=1  OutputSizes=1
  Data Store Write6 : DataStoreWrite  DataStoreName=oTilt  DataStoreElements=oTilt.oMot_.oIn_.fOmegaEObserverRaw2_  IndexOptions=Index vector (dialog)  Indices=1  OutputSizes=1
  Data Store Write7 : DataStoreWrite  DataStoreName=oTilt  DataStoreElements=oTilt.oMot_.oIn_.fId_  IndexOptions=Index vector (dialog)  Indices=1  OutputSizes=1
  Data Store Write8 : DataStoreWrite  DataStoreName=oTilt  DataStoreElements=oTilt.oMot_.oIn_.fIq_  IndexOptions=Index vector (dialog)  Indices=1  OutputSizes=1
  Data Store Write9 : DataStoreWrite  DataStoreName=oTilt  DataStoreElements=oTilt.oMot_.oIn_.fIdRefTotal_  IndexOptions=Index vector (dialog)  Indices=1  OutputSizes=1
  wires:
  Data Store Read23/1 -> Data Store Write24/1
  Data Store Read18/1 -> Data Store Write19/1
  Data Store Read13/1 -> Data Store Write14/1
  Data Store Read12/1 -> Data Store Write13/1
  Data Store Read20/1 -> Data Store Write21/1
  Data Store Read17/1 -> Data Store Write18/1
  Data Store Read19/1 -> Data Store Write20/1
  Data Store Read22/1 -> Data Store Write23/1
  Data Store Read1/1 -> Data Store Write2/1
  Data Store Read6/1 -> Data Store Write7/1
  Data Store Read3/1 -> Data Store Write4/1
  Data Store Read4/1 -> Data Store Write5/1
  Data Store Read7/1 -> Data Store Write8/1
  Data Store Read14/1 -> Data Store Write15/1
  Data Store Read5/1 -> Data Store Write6/1
  Data Store Read21/1 -> Data Store Write22/1
  Data Store Read11/1 -> Data Store Write12/1
  Data Store Read/1 -> Data Store Write1/1
  Constant/1 -> Data Store Write/1
  Data Store Read16/1 -> Data Store Write17/1
  Data Store Read2/1 -> Data Store Write3/1
  Data Store Read15/1 -> Data Store Write16/1
  Data Store Read10/1 -> Data Store Write11/1
  Data Store Read9/1 -> Data Store Write10/1
  Data Store Read8/1 -> Data Store Write9/1

== system Target_Control_System/Target_Control_System/InterruptFunction/tiltMotor_isrSchedule ==
  FunctionCallScheduleTilt : TriggerPort  TriggerType=function-call  VariantControl=Variant
  Constant : Constant  Value=0  OutDataTypeStr=uint32  SampleTime=-1
  Data Store Read : DataStoreRead  DataStoreName=mdl_suiIsrSmallInvCounter_  IndexOptions=Index vector (dialog)  Indices=1  OutputSizes=1
  Equal : RelationalOperator  Operator===  OutDataTypeStr=boolean  RndMeth=Simplest
  Triggered Subsystem : Subsystem  TreatAsAtomicUnit=on
  Output : Outport
  wires:
  Constant/1 -> Equal/2
  Data Store Read/1 -> Equal/1
  Triggered Subsystem/1(Output) -> Output/1
  Equal/1 -> Triggered Subsystem/Trigger

== system Target_Control_System/Target_Control_System/InterruptFunction/tiltMotor_isrTask ==
  motorIntTaskStep : TriggerPort  TriggerType=function-call  VariantControl=Variant  PortDimensions=1
  Function-Call Generator : simulink/Ports & Subsystems/Function-Call Generator  sample_time=-1  numberOfIterations=1  DisallowWideOutput=off
  Function-Call Split{1..8} (8 alike) : FunctionCallSplit  NumOutputPorts=2
  abcToAlphaBeta : Subsystem  TreatAsAtomicUnit=on
  currentController : Subsystem  TreatAsAtomicUnit=on
  dqTransform : Subsystem  TreatAsAtomicUnit=on
  fluxAngleCalculation : Subsystem  TreatAsAtomicUnit=on
  fluxObserver : Subsystem  Commented=on  TreatAsAtomicUnit=on
  isrStateMachine : Subsystem  TreatAsAtomicUnit=on
  pwmGeneration : Subsystem  TreatAsAtomicUnit=on
  resetFlags : Subsystem  TreatAsAtomicUnit=on
  softCurrentLimiting : Subsystem  Commented=on  TreatAsAtomicUnit=on
  wires:
  Function-Call Split8/2 -> isrStateMachine/Trigger
  Function-Call Split8/1 -> pwmGeneration/Trigger
  Function-Call Split7/2 -> Function-Call Split8/1
  Function-Call Split7/1 -> currentController/Trigger
  Function-Call Split1/2 -> Function-Call Split7/1
  Function-Call Split1/1 -> dqTransform/Trigger
  Function-Call Split6/2 -> Function-Call Split1/1
  Function-Call Split6/1 -> fluxAngleCalculation/Trigger
  Function-Call Split5/2 -> Function-Call Split6/1
  Function-Call Split5/1 -> fluxObserver/Trigger
  Function-Call Split4/2 -> Function-Call Split5/1
  Function-Call Split4/1 -> abcToAlphaBeta/Trigger
  Function-Call Split3/2 -> Function-Call Split4/1
  Function-Call Split3/1 -> softCurrentLimiting/Trigger
  Function-Call Split2/2 -> Function-Call Split3/1
  Function-Call Split2/1 -> resetFlags/Trigger
  Function-Call Generator/1 -> Function-Call Split2/1

== system Target_Control_System/Target_Control_System/InterruptFunction/tiltMotor_setPwm ==
  setPwmDuty : TriggerPort  TriggerType=function-call  VariantControl=Variant
  Data Store Read1 : DataStoreRead  DataStoreName=oTilt  DataStoreElements=oTilt.oIsr_.oState_.iPwmUpdated_  IndexOptions=Index vector (dialog)  Indices=1  OutputSizes=1
  ModelSourceFPGATilt : Subsystem  Variant=on
  NOT : Logic  Operator=NOT  AllPortsSameDT=off  OutDataTypeStr=boolean
  Subsystem : Subsystem
  wires:
  NOT/1 -> Subsystem/Enable
  Data Store Read1/1 -> NOT/1

== system Target_Control_System/Target_Control_System/MainLoop/pitchMotor_mainLoop ==
  Decimation gate for 10 Hz Pitch : Subsystem  TreatAsAtomicUnit=on  SystemSampleTime=1/10
  Decimation gate for 200 Hz Pitch : Subsystem  TreatAsAtomicUnit=on  SystemSampleTime=1/200
  Decimation gate for 5000 Hz Pitch : Subsystem  TreatAsAtomicUnit=on  SystemSampleTime=1/5000
  mainTask_pitch : Subsystem  TreatAsAtomicUnit=on  SystemSampleTime=5e-5
  Vabc_pump_pwm_ticks : Outport
  wires:
  mainTask_pitch/1(Out1) -> Vabc_pump_pwm_ticks/1  "pitchMotor_PWMticks"

== system Target_Control_System/Target_Control_System/MainLoop/propMotor_mainLoop ==
  Decimation gate A for 200 Hz Prop : Subsystem  TreatAsAtomicUnit=on  SystemSampleTime=1/200
  Decimation gate for 5000 Hz Prop : Subsystem  TreatAsAtomicUnit=on  SystemSampleTime=1/5000
  motorStateMachineLogic(&oProp) : Subsystem  TreatAsAtomicUnit=on  SystemSampleTime=0.01*(TARGET_CODE_GEN==0)+0.1*(TARGET_CODE_GEN==1)
  motorTaskMainFastStep(&oProp) : Subsystem  TreatAsAtomicUnit=on  SystemSampleTime=1.25E-5
  Out1 : Outport
  wires:
  motorTaskMainFastStep(&oProp)/1(Motor) -> Out1/1  "propMotor_PWMticks"

== system Target_Control_System/Target_Control_System/MainLoop/pumpMotor_mainLoop ==
  Decimation gate A for 200 Hz Pump : Subsystem  TreatAsAtomicUnit=on  SystemSampleTime=1/200
  Decimation gate for 5000 Hz Pump : Subsystem  TreatAsAtomicUnit=on  SystemSampleTime=1/5000
  motorStateMachineLogic(&oPump) : Subsystem  TreatAsAtomicUnit=on  SystemSampleTime=0.01*(TARGET_CODE_GEN==0)+0.1*(TARGET_CODE_GEN==1)
  motorTaskMainFastStep(&oPump) : Subsystem  TreatAsAtomicUnit=on  SystemSampleTime=2.5E-5
  Vabc_pump_pwm_ticks : Outport
  wires:
  motorTaskMainFastStep(&oPump)/1(Motor) -> Vabc_pump_pwm_ticks/1  "pumpMotor_PWMticks"

== system Target_Control_System/Target_Control_System/MainLoop/tiltMotor_mainLoop ==
  Decimation gate for 10 Hz Tilt : Subsystem  TreatAsAtomicUnit=on  SystemSampleTime=1/10
  Decimation gate for 200 Hz Tilt : Subsystem  TreatAsAtomicUnit=on  SystemSampleTime=1/200
  Decimation gate for 5000 Hz Tilt : Subsystem  TreatAsAtomicUnit=on  SystemSampleTime=1/5000
  mainTask_tilt : Subsystem  TreatAsAtomicUnit=on  SystemSampleTime=5e-5
  Vabc_pump_pwm_ticks : Outport
  wires:
  mainTask_tilt/1(Out1) -> Vabc_pump_pwm_ticks/1  "tiltMotor_PWMticks"

== system Target_Control_System/Target_Control_System/ModelSource/DoNotIncludeCustomCode ==

== system Target_Control_System/Target_Control_System/ModelSource/IncludeCustomCode ==
  Model Source : Subsystem  mask(Model Source){ShowInLibBrowser=0}
      mask prompts: ShowInLibBrowser "Simulink:masks:CustCodeMaskParam1_MP"
      settings: CopyFcn=cccopyfcn(gcb)  OpenFcn=ccopenfcn('Model Source')
      mask Help: eval('feval(''rtwprivate'',''rtwhelpview'',''rtw_model_source_block'')');
      mask DialogControl ShowInLibBrowser Prompt: Mask Parameter 1:
      mask Display: disp('Model\nSource');
